simulink model "twolink_observer"  (R2014a)
settings: Solver=ode45  StartTime=0.0  StopTime=5.0  RelTol=1e-3
settings Model: Creator=Serhat  LastModifiedBy=Serhat

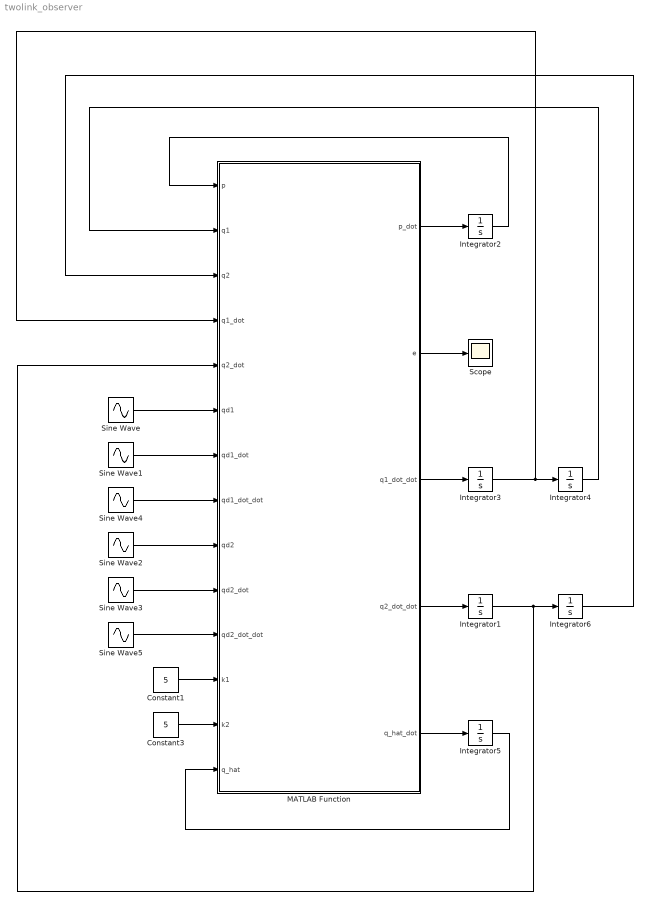
== system twolink_observer ==
  Constant1 : Constant  Value=5
  Constant3 : Constant  Value=5
  Integrator{1..6} (6 alike) : Integrator  InitialCondition=10
  MATLAB Function : MATLAB Function  TreatAsAtomicUnit=on
  Scope : Scope
  Sine Wave : Sin  SampleTime=0
  Sine Wave1 : Sin  Phase=pi/2  SampleTime=0
  Sine Wave2 : Sin  SampleTime=0
  Sine Wave3 : Sin  Phase=pi/2  SampleTime=0
  Sine Wave4 : Sin  Phase=pi  SampleTime=0
  Sine Wave5 : Sin  Phase=pi  SampleTime=0
  wires:
  Sine Wave/1 -> MATLAB Function/6(qd1)
  Sine Wave1/1 -> MATLAB Function/7(qd1_dot)
  Sine Wave2/1 -> MATLAB Function/9(qd2)
  Sine Wave3/1 -> MATLAB Function/10(qd2_dot)
  MATLAB Function/2(e) -> Scope/1
  Sine Wave4/1 -> MATLAB Function/8(qd1_dot_dot)
  Sine Wave5/1 -> MATLAB Function/11(qd2_dot_dot)
  Constant1/1 -> MATLAB Function/12(k1)
  Constant3/1 -> MATLAB Function/13(k2)
  MATLAB Function/1(p_dot) -> Integrator2/1
  Integrator2/1 -> MATLAB Function/1(p)
  MATLAB Function/5(q_hat_dot) -> Integrator5/1
  Integrator5/1 -> MATLAB Function/14(q_hat)
  MATLAB Function/4(q2_dot_dot) -> Integrator1/1
  MATLAB Function/3(q1_dot_dot) -> Integrator3/1
  Integrator4/1 -> MATLAB Function/2(q1)
  Integrator6/1 -> MATLAB Function/3(q2)
  Integrator3/1 -> MATLAB Function/4(q1_dot), Integrator4/1
  Integrator1/1 -> MATLAB Function/5(q2_dot), Integrator6/1

== matlab function twolink_observer/MATLAB Function ==
  data: p input; p_dot output; q1 input; q2 input; q1_dot input; q2_dot input; qd1 input; qd1_dot input; qd1_dot_dot input; qd2 input; qd2_dot input; qd2_dot_dot input; k1 input; k2 input; e output; q1_dot_dot output; q2_dot_dot output; q_hat_dot output; q_hat input
function [p_dot,e , q1_dot_dot, q2_dot_dot, q_hat_dot]= fcn(p, q1, q2, q1_dot, q2_dot,  qd1, qd1_dot, qd1_dot_dot, qd2, qd2_dot, qd2_dot_dot, k1, k2, q_hat)
%#codegen

g = 9.8;

% Inertia Matrix
m1 = 1;
m2 = 1;

l1 = 0.40;
l2 = 0.40;

M12 = m2*l1*l2*cos(q2) + m2*(l2^2);
M21 = M12;
M22 = m2*(l2^2);
M11 = M22;

M = [ M11 M12 ; M21 M22];


% Centripedal Matrix
h = m2*l1*l2*sin(q2);

V11 = -h*q2_dot;
V12 = -h*q1_dot-h*q2_dot;
V21 = h*q1_dot;
V22 = 0;

V = [V11 V12; V21 V22 ];


% F
F1 = V(1)*q1_dot;
F2 = V(2)*q2_dot;

F = [ F1;  F2];


% Gravity
G1 = m1*l1*cos(q1) + m2*g*(l2*cos(q1+q2) + l1*cos(q1)); %???
G2 = m2*l2*g*cos(q1+q2);

G = [ G1; G2];


% Disturbance?
Td1 = k1*sign(q1_dot);
Td2 = k2 *sign(q2_dot);

Td = [ Td1; Td2];


% error & auxilary function
a = 3;
k = 100;

e11 = q1 - qd1;
e12 = q2 - qd2;

e = [e11; e12];

ed11 = q1_dot - qd1_dot;
ed12 = q2_dot - qd2_dot;
e_dot = [ed11; ed12];


q = [q1; q2];
q_dot = [q1_dot; q2_dot];
qd = [qd1; qd2];
qd_dot = [qd1_dot; qd2_dot];
qd_dot_dot = [qd1_dot_dot; qd2_dot_dot];



q_tilda = q - q_hat;
p_dot = -q + (a + 1)*q_tilda;
q_hat_dot = -q + (a+1)*q_tilda + p;
